simulink model "EV_Model_2022a"  (R2022a)
settings: Solver=FixedStepAuto  StartTime=0.0  StopTime=100  FixedStep=0.01  RelTol=1e-3
model workspace (MAT data in the model file):
  CLTC = [0 1 2 3 4 5 6 7 8 9 10 11 ... (3602 elements, 1801x2)]
  NETC = [0 1 2 3 4 5 6 7 8 9 10 11 ... (2362 elements, 1181x2)]
values from neighbouring files (symbols this model uses):
  Area = 2.3    [Data.m]
  BattNp = 40    [Data.m]
  BattNs = 100    [Data.m]
  Cd = 0.28    [Data.m]
  CellCap = 4.5    [Data.m]
  CellResis = 0.003    [Data.m]
  f = 0.01    [Data.m]
  g = 9.8    [Data.m]
  GearEff = 0.97    [Data.m]
  GearRto = 9.7    [Data.m]
  Grad = 0    [Data.m]
  MotDrvCrv_1X_rpm = [1000 2000 3000 4000 5000 6000 7000 8000 9000 10000 12000 13000 14000 15000 16000]    [Data.m]
  MotDrvCrv_1Y_Tq = [390 390 390 389 311 259 222 195 173 156 142 130 120 111 104]    [Data.m]
  MotEffMap_2X_rpm = [472 944 1416 1888 2360 2832 3304 3776 4248 4720 5192 5664 6136 6608 7080 7552 8024 8496 8968 9440 9912 10384 10856 11328 11800 12272 12744 13216 13688 14160 14632 15104 15500]    [Data.m]
  MotEffMap_2Y_Nm = [0 10 20 30 40 50 60 70 80 90 100 110 120 130 140 150 160 170 180 190 200 210 220 230 240 250 260 270 280 290 310 320 330 340]    [Data.m]
  MotEffMap_2Z_pct = [ [67.63 68.67 69.65 70.57 71.41 72.20 72.92 73.57 74.16 74.68 75.14 75.53 75.86 76.12 76.31 76.44 76.51 76.51 76.44 76.31 76.12 75.86 75.53 75.14 74.68 74.16 73.57 72.92 72.20 71.41 70.57 69.65 68.67 67.63]; [68.87 70.13 71.31 72.41 73.43 74.38 75.24 76.03 76.74 77.36 77.91 78.39 78.78 79.09 79.33 79.49 79.57 79.57 79.49 79.33 79.09 78.78 78.39 77.91 77.36 76.74 76.03 75.24 74.38 73.43 72.41 71.3 ...(+6434 chars)    [Data.m]
  MotGenCrv_1X_rpm = MotDrvCrv_1X_rpm    [Data.m]
  MotGenCrv_1Y_Tq = -1*MotDrvCrv_1Y_Tq    [Data.m]
  OCV_1X_pct = [0, 100]    [Data.m]
  OCV_1Y_v = [3.0, 4.2]    [Data.m]
  RotCoeff = 0.05    [Data.m]
  SOCIni = 95    [Data.m]
  SOCMin = 5    [Data.m]
  vhemass = 1500    [Data.m]
  WhlRollRads = 0.327    [Data.m]
libraries: simulink x2, slpidlib x1
settings Model: Creator=bingtao.hu  LastModifiedBy=bingtao.hu
settings ModelReferenceCC: EnableRefExpFcnMdlSchedulingChecks=off
settings RTWCC: Description=Generic Real-Time Target

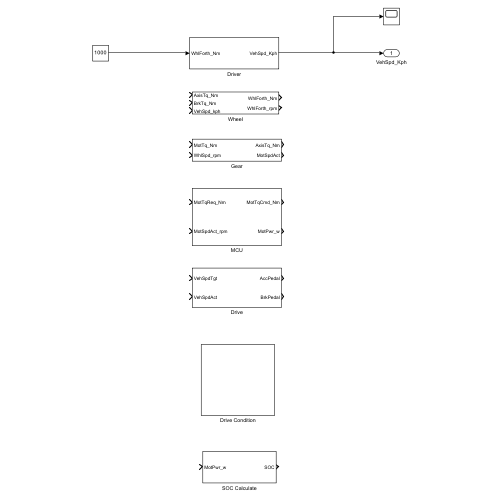
[thumbnail: Simulink's stored preview of the top-level diagram]
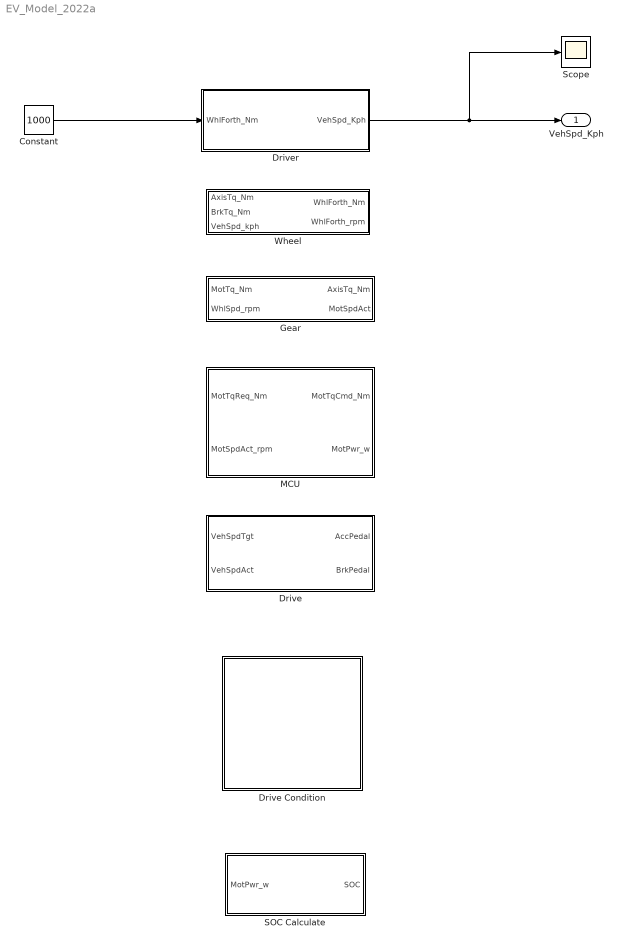
== system EV_Model_2022a ==
  Constant : Constant  Value=1000
  Drive : Subsystem
  Drive Condition : Subsystem
  Driver : Subsystem
  Gear : Subsystem
  MCU : Subsystem
  SOC Calculate : Subsystem
  Scope : Scope
  Wheel : Subsystem
  VehSpd_Kph : Outport
  wires:
  Constant/1 -> Driver/1(WhlForth_Nm)
  Driver/1(VehSpd_Kph) -> Scope/1, VehSpd_Kph/1

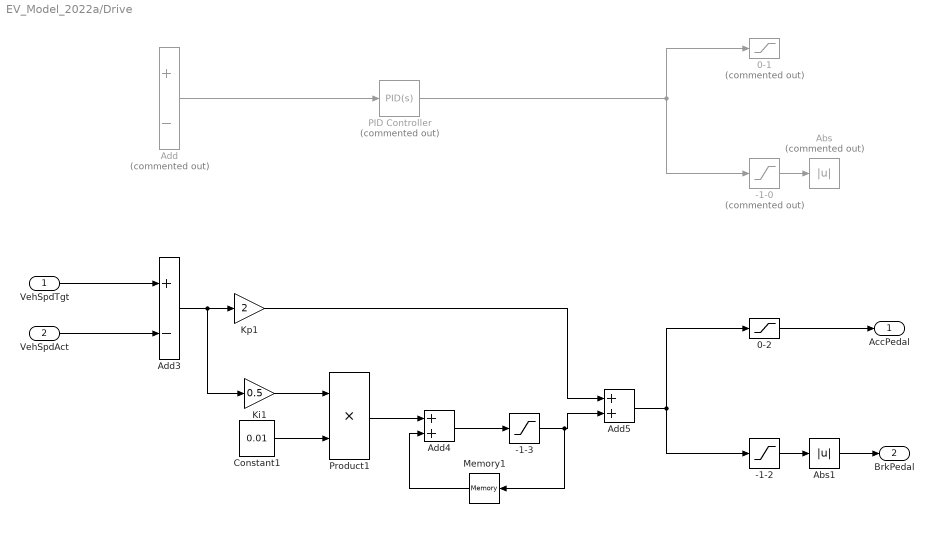
== system EV_Model_2022a/Drive ==
  VehSpdTgt : Inport
  VehSpdAct : Inport  Port=2
  -1-0 : Saturate  Commented=on  UpperLimit=0  LowerLimit=-1
  -1-2 : Saturate  UpperLimit=0  LowerLimit=-1
  -1-3 : Saturate  UpperLimit=1  LowerLimit=-1
  0-1 : Saturate  Commented=on  UpperLimit=1  LowerLimit=0
  0-2 : Saturate  UpperLimit=1  LowerLimit=0
  Abs : Abs  Commented=on  SaturateOnIntegerOverflow=off
  Abs1 : Abs  SaturateOnIntegerOverflow=off
  Add : Sum  Commented=on  Inputs=+-
  Add3 : Sum  Inputs=+-
  Add4 : Sum
  Add5 : Sum
  Constant1 : Constant  Value=0.01
  Ki1 : Gain  Gain=0.5
  Kp1 : Gain  Gain=2
  Memory1 : Memory
  PID Controller : slpidlib/PID Controller  Commented=on  Controller=PID  Form=Parallel  TimeDomain=Continuous-time  UseExternalTs=off  SampleTime=-1  IntegratorMethod=Forward Euler  FilterMethod=Forward Euler  ControllerParametersSource=internal  P=1  I=1  UseKiTs=off  D=0  N=100  UseFilter=on  TunerSelectOption=Transfer Function Based (PID Tuner App)  InitialConditionSource=internal  InitialConditionForIntegrator=0  InitialConditionForFilter=0  DifferentiatorICPrevScaledInput=0  ExternalReset=none  TrackingMode=off  Kt=1  LimitOutput=off  SatLimitsSource=internal  UpperSaturationLimit=inf  LowerSaturationLimit=-inf  LinearizeAsGain=on  AntiWindupMode=none  Kb=1  POutMin=[]  POutMax=[]  IOutMin=[]  IOutMax=[]  DOutMin=[]  DOutMax=[]  NOutMin=[]  NOutMax=[]  SumOutMin=[]  SumOutMax=[]  SaturationOutMin=[]  SaturationOutMax=[]  PParamMin=[]  PParamMax=[]  IParamMin=[]  IParamMax=[]  DParamMin=[]  DParamMax=[]  NParamMin=[]  NParamMax=[]  KbParamMin=[]  KbParamMax=[]  KtParamMin=[]  KtParamMax=[]  KbOutMin=[]  KbOutMax=[]  KtOutMin=[]  KtOutMax=[]  IntegratorOutMin=[]  IntegratorOutMax=[]  FilterOutMin=[]  FilterOutMax=[]  SumI1OutMin=[]  SumI1OutMax=[]  SumI2OutMin=[]  SumI2OutMax=[]  SumI3OutMin=[]  SumI3OutMax=[]  SumI4OutMin=[]  SumI4OutMax=[]  SumDOutMin=[]  SumDOutMax=[]  DifferentiatorOutMin=[]  DifferentiatorOutMax=[]  FilterDiffOutCoefMin=[]  FilterDiffOutCoefMax=[]  ReciprocalOutMin=[]  ReciprocalOutMax=[]  SumDenOutMin=[]  SumDenOutMax=[]  SumNumOutMin=[]  SumNumOutMax=[]  DivideOutMin=[]  DivideOutMax=[]  UdiffTsProdOutMin=[]  UdiffTsProdOutMax=[]  NTsProdOutMin=[]  NTsProdOutMax=[]  UintegralTsProdOutMin=[]  UintegralTsProdOutMax=[]  UngainTsProdOutMin=[]  UngainTsProdOutMax=[]  IntegratorContinuousStateAttributes=''  IntegratorStateMustResolveToSignalObject=off  IntegratorRTWStateStorageClass=Auto  FilterContinuousStateAttributes=''  FilterStateMustResolveToSignalObject=off  FilterRTWStateStorageClass=Auto  ParallelPVariant=InternalParameters  IdealPVariant=Disabled  IVariant=InternalParameters  DVariant=InternalParameters  IntegratorVariant=Continuous  SatVariant=Disabled  AWVariant=Passthrough  PCopyVariant=Disabled  TRVariant=Disabled  FdbkBlocksVariant=Forward  IdealPFdbkVariant=Disabled  SatFdbkVariant=Disabled  DerivativeFilterVariant=ContFilter  NVariant=InternalParameters  NCopyVariant=Disabled  FilterICVariant=InternalICsFilter  IntegratorICVariant=InternalICs  ExternalResetVariant=Disabled  TRSumVariant=Passthrough  SumFdbkVariant=Disabled  SumVariant=Sum_PID  TsampFilterVariant=InternalTs  TsampNgainVariant=Passthrough  TsampIntegralVariant=Disabled_SignalSpec  ExternalSaturationOutDataTypeStr=Inherit: Same as second input
  Product1 : Product
  AccPedal : Outport
  BrkPedal : Outport  Port=2
  wires:
  -1-0/1 -> Abs/1
  Add/1 -> PID Controller/1
  PID Controller/1 -> -1-0/1, 0-1/1
  -1-3/1 -> Memory1/1, Add5/2
  Add4/1 -> -1-3/1
  Add5/1 -> 0-2/1, -1-2/1
  Ki1/1 -> Product1/1
  Constant1/1 -> Product1/2
  Product1/1 -> Add4/1
  Memory1/1 -> Add4/2
  0-2/1 -> AccPedal/1
  VehSpdTgt/1 -> Add3/1
  Abs1/1 -> BrkPedal/1
  -1-2/1 -> Abs1/1
  Kp1/1 -> Add5/1
  Add3/1 -> Ki1/1, Kp1/1
  VehSpdAct/1 -> Add3/2

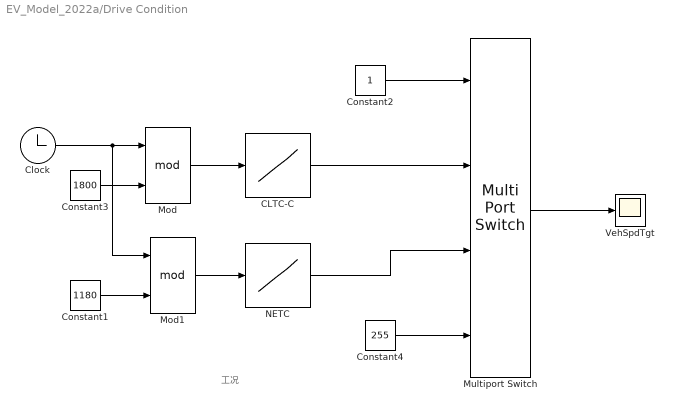
== system EV_Model_2022a/Drive Condition ==
  note: 工况
  CLTC-C : Lookup_n-D  NumberOfTableDimensions=1  BreakpointsForDimension1=CLTC(:,1)  Table=CLTC(:,2)  InternalRulePriority=Speed  RndMeth=Simplest
  Clock : Clock
  Constant1 : Constant  Value=1180
  Constant2 : Constant
  Constant3 : Constant  Value=1800
  Constant4 : Constant  Value=255
  Mod : Math  Operator=mod
  Mod1 : Math  Operator=mod
  Multiport Switch : MultiPortSwitch  SaturateOnIntegerOverflow=off  InputSameDT=off
  NETC : Lookup_n-D  NumberOfTableDimensions=1  BreakpointsForDimension1=NETC(:,1)  Table=NETC(:,2)  InternalRulePriority=Speed  RndMeth=Simplest
  VehSpdTgt : Scope
  wires:
  Constant1/1 -> Mod1/2
  Mod/1 -> CLTC-C/1
  Multiport Switch/1 -> VehSpdTgt/1
  Clock/1 -> Mod1/1, Mod/1
  Constant3/1 -> Mod/2
  Mod1/1 -> NETC/1
  CLTC-C/1 -> Multiport Switch/2
  Constant4/1 -> Multiport Switch/4
  Constant2/1 -> Multiport Switch/1
  NETC/1 -> Multiport Switch/3

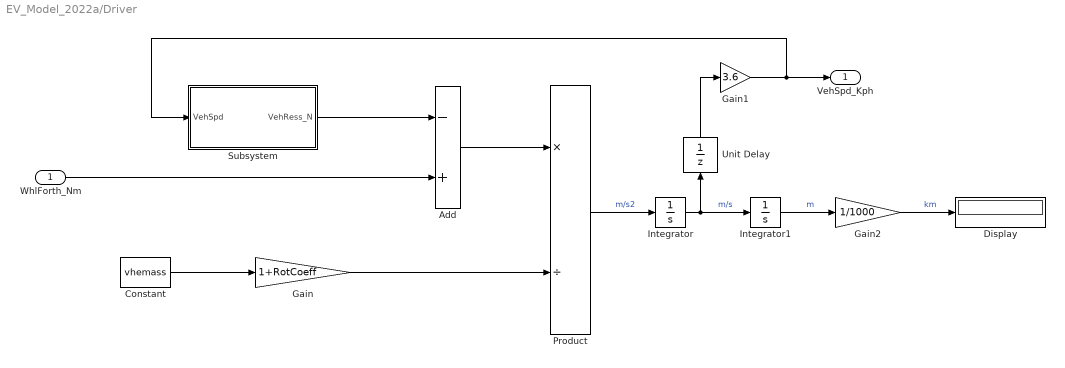
== system EV_Model_2022a/Driver ==
  WhlForth_Nm : Inport
  Add : Sum  Inputs=-+
  Constant : Constant  Value=vhemass
  Display : Display
  Gain : Gain  Gain=1+RotCoeff
  Gain1 : Gain  Gain=3.6
  Gain2 : Gain  Gain=1/1000
  Integrator : Integrator
  Integrator1 : Integrator
  Product : Product  Inputs=*/
  Subsystem : Subsystem
  Unit Delay : UnitDelay  SampleTime=-1  HasFrameUpgradeWarning=on
  VehSpd_Kph : Outport
  wires:
  WhlForth_Nm/1 -> Add/2
  Add/1 -> Product/1
  Gain1/1 -> VehSpd_Kph/1, Subsystem/1(VehSpd)
  Gain/1 -> Product/2
  Gain2/1 -> Display/1  "km"
  Subsystem/1(VehRess_N) -> Add/1
  Constant/1 -> Gain/1
  Product/1 -> Integrator/1  "m/s2"
  Integrator1/1 -> Gain2/1  "m"
  Integrator/1 -> Integrator1/1, Unit Delay/1  "m/s"
  Unit Delay/1 -> Gain1/1

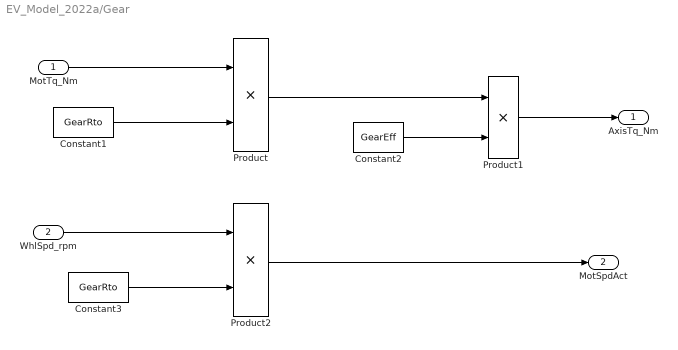
== system EV_Model_2022a/Gear ==
  MotTq_Nm : Inport
  WhlSpd_rpm : Inport  Port=2
  Constant1 : Constant  Value=GearRto
  Constant2 : Constant  Value=GearEff
  Constant3 : Constant  Value=GearRto
  Product : Product
  Product1 : Product
  Product2 : Product
  AxisTq_Nm : Outport
  MotSpdAct : Outport  Port=2
  wires:
  WhlSpd_rpm/1 -> Product2/1
  Constant1/1 -> Product/2
  Product/1 -> Product1/1
  Constant3/1 -> Product2/2
  Product1/1 -> AxisTq_Nm/1
  Constant2/1 -> Product1/2
  Product2/1 -> MotSpdAct/1
  MotTq_Nm/1 -> Product/1

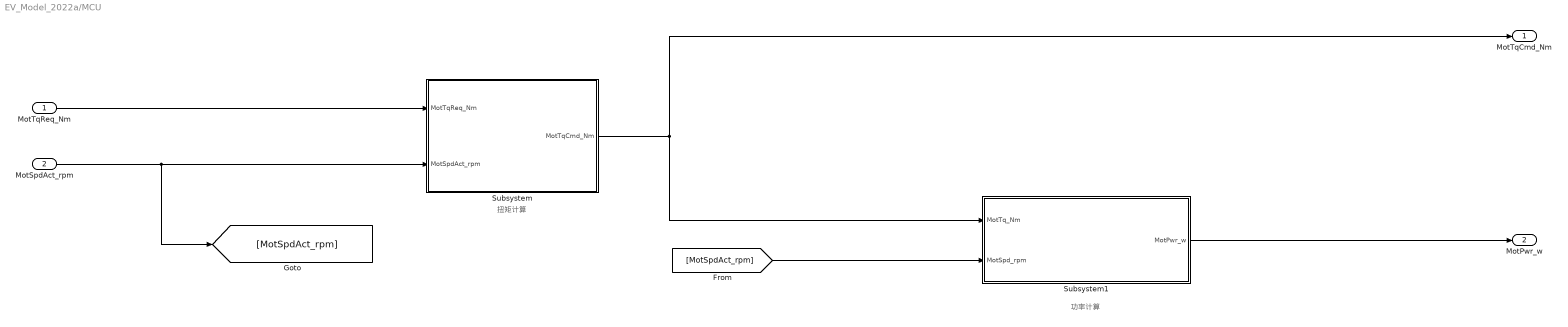
== system EV_Model_2022a/MCU ==
  note: 功率计算
  note: 扭矩计算
  MotTqReq_Nm : Inport
  MotSpdAct_rpm : Inport  Port=2
  Subsystem : Subsystem
  Subsystem1 : Subsystem
  MotTqCmd_Nm : Outport
  MotPwr_w : Outport  Port=2
  wires:
  Subsystem1/1(MotPwr_w) -> MotPwr_w/1
  MotSpdAct_rpm/1 -> Subsystem/2(MotSpdAct_rpm), [MotSpdAct_rpm]
  Subsystem/1(MotTqCmd_Nm) -> MotTqCmd_Nm/1, Subsystem1/1(MotTq_Nm)
  MotTqReq_Nm/1 -> Subsystem/1(MotTqReq_Nm)
  [MotSpdAct_rpm] -> Subsystem1/2(MotSpd_rpm)

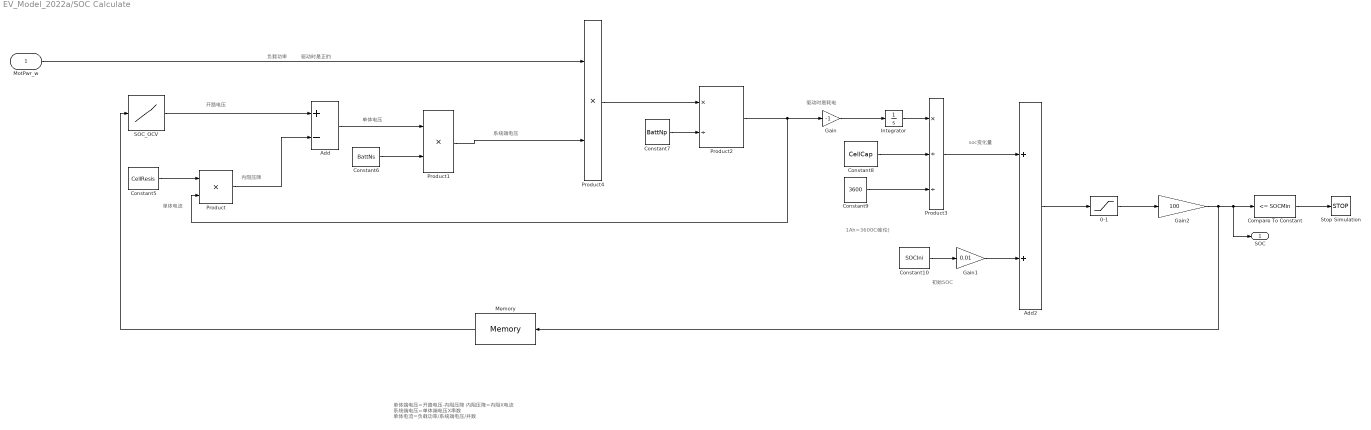
== system EV_Model_2022a/SOC Calculate ==
  note: 驱动时是耗电
  note: 初始SOC
  note: soc变化量
  note: 1Ah=3600C(库伦)
  note: 驱动时是正的
  note: 开路电压
  note: 负载功率
  note: 单体电压
  note: 系统端电压
  note: 内阻压降
  note: 单体电流
  note: 单体端电压=开路电压-内阻压降
      | 内阻压降=内阻X电流
      | 系统端电压=单体端电压X串数
      | 单体电流=负载功率/系统端电压/并数
  MotPwr_w : Inport
  0-1 : Saturate  UpperLimit=1  LowerLimit=0
  Add : Sum  Inputs=+-
  Add2 : Sum
  Compare To Constant : simulink/Logic and Bit Operations/Compare To Constant  relop=<=  const=SOCMin  OutDataTypeStr=boolean
  Constant10 : Constant  Value=SOCIni
  Constant5 : Constant  Value=CellResis
  Constant6 : Constant  Value=BattNs
  Constant7 : Constant  Value=BattNp
  Constant8 : Constant  Value=CellCap
  Constant9 : Constant  Value=3600
  Gain : Gain  Gain=-1
  Gain1 : Gain  Gain=0.01
  Gain2 : Gain  Gain=100
  Integrator : Integrator
  Memory : Memory
  Product : Product
  Product1 : Product
  Product2 : Product  Inputs=*/
  Product3 : Product  Inputs=*//
  Product4 : Product
  SOC_OCV : Lookup_n-D  NumberOfTableDimensions=1  BreakpointsForDimension1=OCV_1X_pct  Table=OCV_1Y_v  InternalRulePriority=Speed  RndMeth=Simplest
  Stop Simulation : Stop
  SOC : Outport
  wires:
  Compare To Constant/1 -> Stop Simulation/1
  Product2/1 -> Product/2, Gain/1
  Product3/1 -> Add2/1
  Product/1 -> Add/2
  Constant9/1 -> Product3/3
  Constant10/1 -> Gain1/1
  Constant5/1 -> Product/1
  Product4/1 -> Product2/1
  Add/1 -> Product1/1
  Gain1/1 -> Add2/2
  Add2/1 -> 0-1/1
  Gain/1 -> Integrator/1
  Integrator/1 -> Product3/1
  Constant6/1 -> Product1/2
  Gain2/1 -> SOC/1, Compare To Constant/1, Memory/1
  Product1/1 -> Product4/2
  Memory/1 -> SOC_OCV/1
  0-1/1 -> Gain2/1
  MotPwr_w/1 -> Product4/1
  SOC_OCV/1 -> Add/1
  Constant7/1 -> Product2/2
  Constant8/1 -> Product3/2

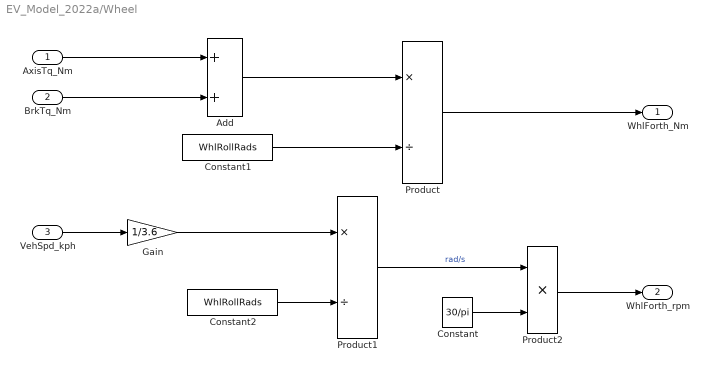
== system EV_Model_2022a/Wheel ==
  AxisTq_Nm : Inport
  BrkTq_Nm : Inport  Port=2
  VehSpd_kph : Inport  Port=3
  Add : Sum
  Constant : Constant  Value=30/pi
  Constant1 : Constant  Value=WhlRollRads
  Constant2 : Constant  Value=WhlRollRads
  Gain : Gain  Gain=1/3.6
  Product : Product  Inputs=*/
  Product1 : Product  Inputs=*/
  Product2 : Product
  WhlForth_Nm : Outport
  WhlForth_rpm : Outport  Port=2
  wires:
  BrkTq_Nm/1 -> Add/2
  AxisTq_Nm/1 -> Add/1
  Product/1 -> WhlForth_Nm/1
  Add/1 -> Product/1
  Constant1/1 -> Product/2
  VehSpd_kph/1 -> Gain/1
  Gain/1 -> Product1/1
  Constant2/1 -> Product1/2
  Product1/1 -> Product2/1  "rad/s"
  Constant/1 -> Product2/2
  Product2/1 -> WhlForth_rpm/1

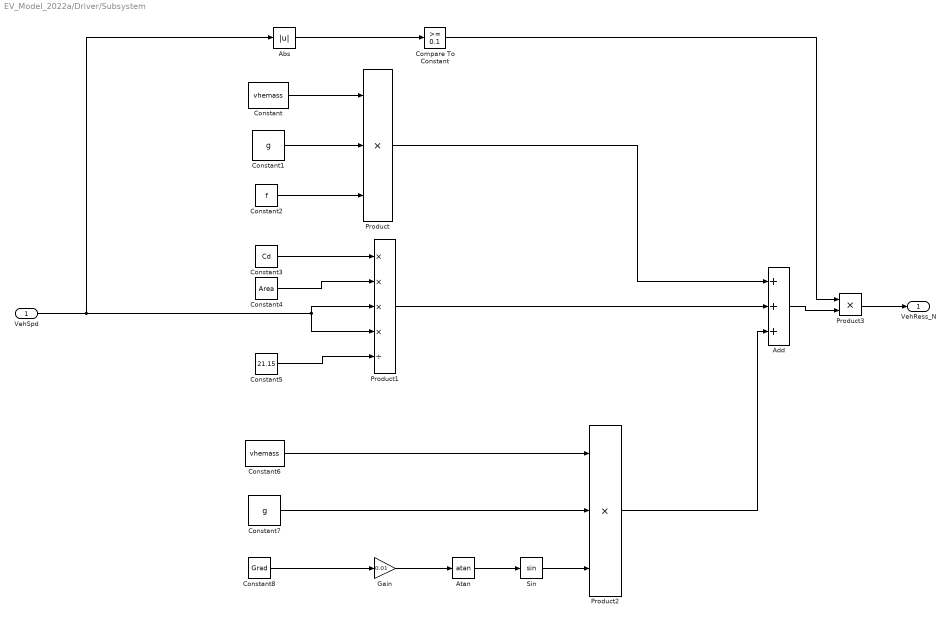
== system EV_Model_2022a/Driver/Subsystem ==
  VehSpd : Inport
  Abs : Abs  SaturateOnIntegerOverflow=off
  Add : Sum  Inputs=+++
  Atan : Trigonometry  Operator=atan
  Compare To Constant : simulink/Logic and Bit Operations/Compare To Constant  relop=>=  const=0.1  OutDataTypeStr=boolean
  Constant : Constant  Value=vhemass
  Constant1 : Constant  Value=g
  Constant2 : Constant  Value=f
  Constant3 : Constant  Value=Cd
  Constant4 : Constant  Value=Area
  Constant5 : Constant  Value=21.15
  Constant6 : Constant  Value=vhemass
  Constant7 : Constant  Value=g
  Constant8 : Constant  Value=Grad
  Gain : Gain  Gain=0.01
  Product : Product  Inputs=3
  Product1 : Product  Inputs=****/
  Product2 : Product  Inputs=3
  Product3 : Product
  Sin : Trigonometry
  VehRess_N : Outport
  wires:
  Constant5/1 -> Product1/5
  VehSpd/1 -> Abs/1, Product1/3, Product1/4
  Constant7/1 -> Product2/2
  Constant/1 -> Product/1
  Gain/1 -> Atan/1
  Constant3/1 -> Product1/1
  Constant4/1 -> Product1/2
  Atan/1 -> Sin/1
  Product2/1 -> Add/3
  Product1/1 -> Add/2
  Sin/1 -> Product2/3
  Constant6/1 -> Product2/1
  Product/1 -> Add/1
  Constant8/1 -> Gain/1
  Constant1/1 -> Product/2
  Constant2/1 -> Product/3
  Abs/1 -> Compare To Constant/1
  Compare To Constant/1 -> Product3/1
  Add/1 -> Product3/2
  Product3/1 -> VehRess_N/1

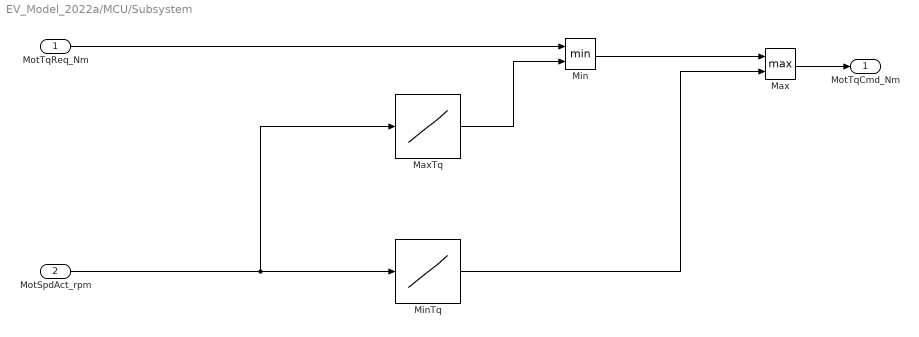
== system EV_Model_2022a/MCU/Subsystem ==
  MotTqReq_Nm : Inport
  MotSpdAct_rpm : Inport  Port=2
  Max : MinMax  Function=max  Inputs=2
  MaxTq : Lookup_n-D  NumberOfTableDimensions=1  BreakpointsForDimension1=MotDrvCrv_1X_rpm  Table=MotDrvCrv_1Y_Tq  ExtrapMethod=Clip  UseLastTableValue=on  InternalRulePriority=Speed  RndMeth=Simplest
  Min : MinMax  Inputs=2
  MinTq : Lookup_n-D  NumberOfTableDimensions=1  BreakpointsForDimension1=MotGenCrv_1X_rpm  Table=MotGenCrv_1Y_Tq  ExtrapMethod=Clip  UseLastTableValue=on  InternalRulePriority=Speed  RndMeth=Simplest
  MotTqCmd_Nm : Outport
  wires:
  Max/1 -> MotTqCmd_Nm/1
  MaxTq/1 -> Min/2
  MinTq/1 -> Max/2
  Min/1 -> Max/1
  MotSpdAct_rpm/1 -> MaxTq/1, MinTq/1
  MotTqReq_Nm/1 -> Min/1

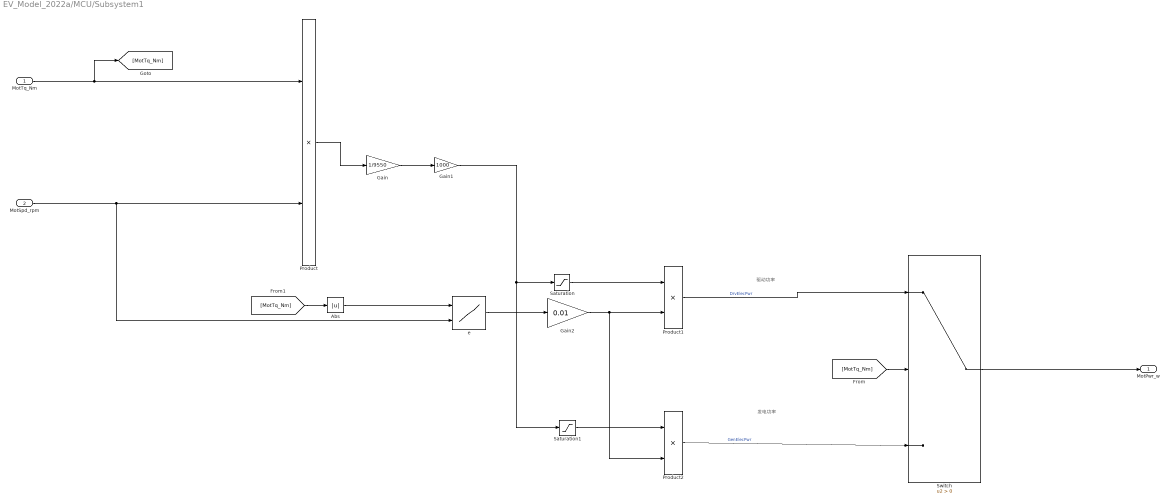
== system EV_Model_2022a/MCU/Subsystem1 ==
  note: 发电功率
  note: 驱动功率
  MotTq_Nm : Inport
  MotSpd_rpm : Inport  Port=2
  Abs : Abs  SaturateOnIntegerOverflow=off
  Gain : Gain  Gain=1/9550
  Gain1 : Gain  Gain=1000
  Gain2 : Gain  Gain=0.01
  Product : Product
  Product1 : Product
  Product2 : Product
  Saturation : Saturate  UpperLimit=inf  LowerLimit=0
  Saturation1 : Saturate  UpperLimit=0  LowerLimit=-inf
  Switch : Switch  Criteria=u2 > Threshold  SaturateOnIntegerOverflow=off  InputSameDT=off
  e : Lookup_n-D  BreakpointsForDimension1=MotEffMap_2X_rpm  BreakpointsForDimension2=MotEffMap_2Y_Nm  Table=MotEffMap_2Z_pct  ExtrapMethod=Clip  UseLastTableValue=on  InternalRulePriority=Speed  RndMeth=Simplest
      settings: InputPortMap=u0,u1
  MotPwr_w : Outport
  wires:
  e/1 -> Gain2/1
  Gain/1 -> Gain1/1
  Gain2/1 -> Product2/2, Product1/2
  Saturation/1 -> Product1/1
  Saturation1/1 -> Product2/1
  MotTq_Nm/1 -> [MotTq_Nm], Product/1
  Product1/1 -> Switch/1  "DrvElecPwr"
  Product/1 -> Gain/1
  Abs/1 -> e/1
  Gain1/1 -> Saturation1/1, Saturation/1
  Product2/1 -> Switch/3  "GenElecPwr"
  MotSpd_rpm/1 -> e/2, Product/2
  Switch/1 -> MotPwr_w/1
  [MotTq_Nm] -> Switch/2
  [MotTq_Nm] -> Abs/1
